simulink model "es5_sim"  (R2023b)
settings: Solver=VariableStepAuto  StartTime=0.0  StopTime=50  RelTol=1e-3
values from neighbouring files (symbols this model uses):
  A3 = J3    [es5.m]
  B3 = double(subs(B_s,[x1,x2,u],[xeq3,ueq]))    [es5.m]
  C3 = double(subs(C_s,[x1,x2,u],[xeq3,ueq]))    [es5.m]
  ueq = 0.5    [es5.m]
  x0 = [10,10]    [es5.m]
  xeq3 = double([xeq_s.x1(3) xeq_s.x2(3)])    [es5.m]
settings Model: Creator=claudio  LastModifiedBy=stefa
settings OptimizationCC: ReuseModelBlockBuffer=off

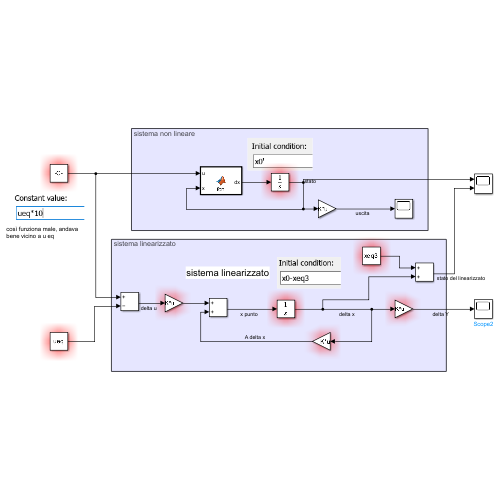
[thumbnail: Simulink's stored preview of the top-level diagram]
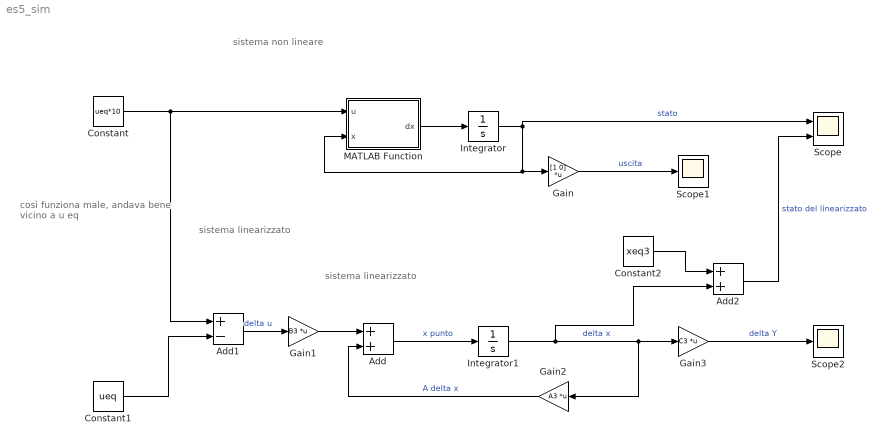
== system es5_sim ==
  note: sistema linearizzato
  note: sistema non lineare
  note: così funziona male, andava bene vicino a u eq
  note: sistema linearizzato
  Add : Sum
  Add1 : Sum  Inputs=+-
  Add2 : Sum
  Constant : Constant  Value=ueq*10
  Constant1 : Constant  Value=ueq
  Constant2 : Constant  Value=xeq3
  Gain : Gain  Gain=[1 0]  Multiplication=Matrix(K*u)
  Gain1 : Gain  Gain=B3  Multiplication=Matrix(K*u)
  Gain2 : Gain  Gain=A3  Multiplication=Matrix(K*u)
  Gain3 : Gain  Gain=C3  Multiplication=Matrix(K*u)
  Integrator : Integrator  InitialCondition=x0'
  Integrator1 : Integrator  InitialCondition=x0-xeq3
  MATLAB Function : MATLAB Function  TreatAsAtomicUnit=on
  Scope : Scope  NumInputPorts=2
  Scope1 : Scope
  Scope2 : Scope
  wires:
  Constant/1 -> Add1/1, MATLAB Function/1(u)
  MATLAB Function/1(dx) -> Integrator/1
  Integrator/1 -> MATLAB Function/2(x), Gain/1, Scope/1  "stato"
  Gain/1 -> Scope1/1  "uscita"
  Gain2/1 -> Add/2  "A delta x"
  Gain1/1 -> Add/1
  Add/1 -> Integrator1/1  "x punto"
  Integrator1/1 -> Add2/2, Gain3/1, Gain2/1  "delta x"
  Add1/1 -> Gain1/1  "delta u"
  Constant1/1 -> Add1/2
  Constant2/1 -> Add2/1
  Add2/1 -> Scope/2  "stato del linearizzato"
  Gain3/1 -> Scope2/1  "delta Y"

== matlab function es5_sim/MATLAB Function ==
  data: u input; dx output; x input
function dx = fcn(u,x)
b=0.1;
a1=0.02; %
a2=0.001; %
k=100; %

%definizione di variabili di tipo simbolico 
%scrivo dx/dt=f(x,u) (in questo caso u=d)
A=x(1);
P=x(2);
dx=[A*(1-A/k)-P*A*a1;-b*P+A*P*a2+u];
